simulink model "S_MTET_2RuleMa_MPPT_CONT_V1"  (R2017a)
settings: Solver=FixedStepDiscrete  StartTime=0.0  StopTime=10.0  RelTol=1e-3
values from neighbouring files (symbols this model uses):
  A = [0 (d-1)/L ... (first row only)    [M_MPPT_CONTROLLERS_SIM_V1.m]
undefined symbols (not defined in the file or in its folder): Down, GPTRIP1SEL, GPTRIP2SEL, TZ1, TZ2, Up
libraries: c2802xlib x3, c2806xlib x2, fuzblock x1
settings Model: ExtModeTrigDuration=8  Creator=dricl  LastModifiedBy=dricl
settings OptimizationCC: DefaultUnderspecifiedDataType=single  PassReuseOutputArgsAs=Individual arguments  MaxStackSize=512
settings DebuggingCC: ParameterTunabilityLossMsg=error
settings HardwareCC: ProdBitPerChar=16  ProdBitPerInt=16  ProdBitPerPointer=32  ProdBitPerSizeT=32  ProdBitPerPtrDiffT=32  ProdLargestAtomicInteger=Integer  ProdLargestAtomicFloat=None  ProdWordSize=16  ProdLongLongMode=on  ProdHWDeviceType=Texas Instruments->C2000
settings SFSimCC: MATLABDynamicMemAlloc=off
settings RTWCC: SystemTargetFile=ert.tlc  HardwareBoard=TI Piccolo F2806x  TLCOptions=-aInlineSetEventsForThisBaseRateFcn=TLC_FALSE -aSuppressMultiTaskScheduler=TLC_FALSE -aRateBasedStepFcn=1  TemplateMakefile=ert_default_tmf  Description=Embedded Coder  Toolchain=Texas Instruments Code Composer Studio v5 (C2000)  CodeExecutionProfiling=on  CodeProfilingSaveOptions=AllData  CodeProfilingInstrumentation=on
settings CodeAppCC: ForceParamTrailComments=on  IgnoreCustomStorageClasses=off  OperatorAnnotations=on  SimulinkDataObjDesc=on  SFDataObjDesc=on  MATLABFcnDesc=on  InsertBlockDesc=on  MATLABSourceComments=on
settings ERTTargetCC: CodeReplacementLibrary=TI C28x  MemSecPackage=tic2000demospkg  MemSecFuncExecute=code_ramfuncs

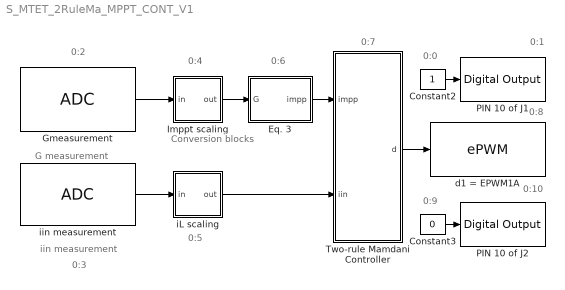
== system S_MTET_2RuleMa_MPPT_CONT_V1 ==
  note: iin measurement
  note: G measurement
  note: Conversion
      | blocks
  note: 0:2
  note: 0:3
  note: 0:4
  note: 0:6
  note: 0:5
  note: 0:7
  note: 0:10
  note: 0:9
  note: 0:0
  note: 0:1
  note: 0:8
  Constant2 : Constant  Priority=1  SampleTime=0.0002
  Constant3 : Constant  Priority=9  Value=0  SampleTime=0.0002
  Eq. 3 : Subsystem  Priority=5  TreatAsAtomicUnit=on
  Gmeasurement : c2802xlib/ADC  Priority=3  ADCModule=1  samplingMode=Single sample mode  ADCResolution=12-bit (Single-ended input)  useSOC1=SOC1  useSOC2=SOC0_SOC1  SOCAcquisitionWindow=7  SOCTriggerSource=ePWM1_ADCSOCA  SOCInterruptTrigger=No ADCINT  Ts=0.0002  dType=uint16  postInterrupt=off  interruptSel=ADCINT1  ADCINTContinuous=on  endma=off  chdma=1  blkParamProc=C2000  conv1=ADCINA1  conv2=ADCINA0 and ADCINB0  conv1_Type4=ADCIN0  conv2_Type4=ADCIN0 and ADCIN1
      settings: SourceProductName=Embedded Coder Support Package for Texas Instruments C2000 Processors
  Imppt scaling : Subsystem  Priority=5  TreatAsAtomicUnit=on
  PIN 10 of J1 : c2806xlib/Digital Output  Priority=2  GPIO_Number=GPIO32~GPIO39  GPIO_Bit0=on  GPIO_BIT0_Toggle=off  GPIO_Bit1=off  GPIO_BIT1_Toggle=off  GPIO_Bit2=off  GPIO_BIT2_Toggle=off  GPIO_Bit3=off  GPIO_BIT3_Toggle=off  GPIO_Bit4=off  GPIO_BIT4_Toggle=off  GPIO_Bit5=off  GPIO_BIT5_Toggle=off  GPIO_Bit6=off  GPIO_BIT6_Toggle=off  GPIO_Bit7=off  GPIO_BIT7_Toggle=off
      settings: SourceProductName=Embedded Coder Support Package for Texas Instruments C2000 Processors  SourceProductBaseCode=TIC2000
  PIN 10 of J2 : c2806xlib/Digital Output  Priority=10  GPIO_Number=GPIO32~GPIO39  GPIO_Bit0=on  GPIO_BIT0_Toggle=off  GPIO_Bit1=off  GPIO_BIT1_Toggle=off  GPIO_Bit2=off  GPIO_BIT2_Toggle=off  GPIO_Bit3=off  GPIO_BIT3_Toggle=off  GPIO_Bit4=off  GPIO_BIT4_Toggle=off  GPIO_Bit5=off  GPIO_BIT5_Toggle=off  GPIO_Bit6=off  GPIO_BIT6_Toggle=off  GPIO_Bit7=off  GPIO_BIT7_Toggle=off
      settings: SourceProductName=Embedded Coder Support Package for Texas Instruments C2000 Processors  SourceProductBaseCode=TIC2000
  Two-rule Mamdani Controller : Subsystem  Priority=7  TreatAsAtomicUnit=on
  d1 = EPWM1A : c2802xlib/ePWM  Priority=8  useModule=ePWM1  ePWMxLINKTBPRD=Not Linked  periodUnits=Clock cycles  timerSource=Specify via dialog  timerPeriod_clk=9000  timerPeriod_sec=0.0001  tbshadow=Counter equals to zero  countingMode=Up-Down  phaseActiveEnable=Disable  phaseDirection=Count down after sync  phaseActive=0  synchronizationEnable=off  dcaevt1Sync=off  dcbevt1Sync=off  synchronizationOption=Disable  clockPrescale=1  HSclockPrescale=1  enswap=off  ePWMxAStatus=on  ePWMxAactionLogic1=Do nothing  ePWMxAactionLogic2=Do nothing  ePWMxAactionLogic3=Clear  ePWMxAactionLogic4=Set  ePWMxAactionLogic5=Do nothing  ePWMxAactionLogic6=Do nothing  ePWMxALoadMode=Load on counter equals to zero (CTR=Zero)  ePWMxACSFenable=off  ePWMxACSFvalue=Forcing disable  ePWMxASFreload=Zero  ePWMxBStatus=off  ePWMxBactionLogic1=Set  ePWMxBactionLogic2=Clear  ePWMxBactionLogic3=Do nothing  ePWMxBactionLogic4=Do nothing  ePWMxBactionLogic5=Clear  ePWMxBactionLogic6=Set  ePWMxBLoadMode=Load on counter equals to zero (CTR=Zero)  ePWMxBCSFenable=off  ePWMxBCSFvalue=Forcing disable  ePWMxBSFreload=Zero  ePWNxBOutWay=off  ePWMxLINKCMPA=Not Linked  CMPAUnits=Clock cycles  CMPASource=Input port  CMPAValue_per=50  CMPAValue_clk=4500  enCMPAshadow=Counter equals to zero  ePWMxLINKCMPB=Not Linked  CMPBUnits=Clock cycles  CMPBSource=Specify via dialog  CMPBValue_per=50  CMPBValue_clk=4500  enCMPBshadow=Counter equals to zero  ePWMxLINKCMPC=Not Linked  CMPCUnits=Clock cycles  CMPCSource=Specify via dialog  CMPCValue_per=50  CMPCValue_clk=32000  enCMPCshadow=Counter equals to zero  ePWMxLINKCMPD=Not Linked  CMPDUnits=Clock cycles  CMPDSource=Specify via dialog  CMPDValue_per=50  CMPDValue_clk=32000  enCMPDshadow=Counter equals to zero  enableDBePWMxA=on  enableDBePWMxB=on  enhalfcycle=off  DBpolarity=Active high complementary (AHC)  DBedgeDelay=Positive  DBSource_ePWMxA=ePWMxA  DBSource_ePWMxB=ePWMxA  DBperiodSource=Specify via dialog  REDperiod=50  FEDperiod=50  adcstartModuleA=on  adcrequestEventA=First event  adcstartEventA=Counter equals to period (CTR=PRD)  adcstartEventA_type2=Digital Compare Module A Event 1 start of conversion (DCAEVT1.soc)  adcstartModuleB=off  adcrequestEventB=First event  adcstartEventB=Counter equals to zero (CTR=Zero)  adcstartEventB_type2=Counter equals to zero (CTR=Zero)  intEn=off  intPrd=First event  intSel=Counter equals to zero (CTR=Zero)  intSel_type2=Counter equals to zero (CTR=Zero)  hrpe=off  enHRPWM=off  HRPWM_LoadMode=Counter equals to period (CTR=PRD)  HRPWM_CTLMode=Duty or Period control mode  HRPWM_EDGMode=Both edge  hrpeb=off  enHRPWMB=off  HRPWM_LoadModeB=Counter equals to zero (CTR=ZERO)  HRPWM_CTLModeB=Duty or Period control mode  HRPWM_EDGModeB=Both edge  enSFO=on  enautoconv=on  chopperEnable=off  chopperFrequency=1  chopperFirstwidth=1  chopperDuty=12.5%  tripZonesource=Specify via dialog  tzselOSHT1=off  tzselOSHT2=off  tzselOSHT3=off  tzselOSHDCAEV1=off  tzselOSHDCBEV1=off  tzselCBC1=off  tzselCBC2=off  tzselCBC3=off  tzselCBCDCAEV2=off  tzselCBCDCBEV2=off  tzselOSHT4=off  tzselOSHT5=off  tzselOSHT6=off  tzselCBC4=off  tzselCBC5=off  tzselCBC6=off  enTzOstIntr=off  enTzCbcIntr=off  enTzDCAEVT1Intr=off  enTzDCAEVT2Intr=off  enTzDCBEVT1Intr=off  enTzDCBEVT2Intr=off  ePWMxAforced=No action  ePWMxBforced=No action  DCAEVT1forced=No action  DCBEVT1forced=No action  DCAEVT2forced=No action  DCBEVT2forced=No action  dcah=Trip Zone 1 input (TZ1)  dcal=Trip Zone 2 input (TZ2)  dcbh=Trip Zone 1 input (TZ1)  dcbl=Trip Zone 2 input (TZ2)  dcah_type2=GPTRIP1SEL/(TZ1)  dcal_type2=GPTRIP2SEL/(TZ2)  dcbh_type2=GPTRIP1SEL/(TZ1)  dcbl_type2=GPTRIP2SEL/(TZ2)  gendcaevt1=Event disabled  gendcaevt2=Event disabled  gendcbevt1=Event disabled  gendcbevt2=Event disabled  dcaevt1src=DCAEVT1 with sync  dcaevt2src=DCAEVT2 with sync  dcbevt1src=DCBEVT1 with sync  dcbevt2src=DCBEVT2 with sync  pulsesel=Counter equals to zero (CTR=Zero)  blankinv=off  blankoffset=0  blankwidth=0  evsrcsel=Filtered version of DCAEVT1 (DCAEVT1FILT)  encape=off  PwmType=C2000
      settings: SourceProductName=Embedded Coder Support Package for Texas Instruments C2000 Processors
  iL scaling : Subsystem  Priority=6  TreatAsAtomicUnit=on
  iin measurement : c2802xlib/ADC  Priority=4  ADCModule=1  samplingMode=Single sample mode  ADCResolution=12-bit (Single-ended input)  useSOC1=SOC2  useSOC2=SOC0_SOC1  SOCAcquisitionWindow=7  SOCTriggerSource=ePWM1_ADCSOCA  SOCInterruptTrigger=No ADCINT  Ts=0.0002  dType=uint16  postInterrupt=off  interruptSel=ADCINT1  ADCINTContinuous=on  endma=off  chdma=1  blkParamProc=C2000  conv1=ADCINA0  conv2=ADCINA0 and ADCINB0  conv1_Type4=ADCIN0  conv2_Type4=ADCIN0 and ADCIN1
      settings: SourceProductName=Embedded Coder Support Package for Texas Instruments C2000 Processors
  wires:
  iL scaling/1(out) -> Two-rule Mamdani Controller/2(iin)
  iin measurement/1 -> iL scaling/1(in)
  Constant2/1 -> PIN 10 of J1/1
  Constant3/1 -> PIN 10 of J2/1
  Two-rule Mamdani Controller/1(d) -> d1 = EPWM1A/1
  Imppt scaling/1(out) -> Eq. 3/1(G)
  Gmeasurement/1 -> Imppt scaling/1(in)
  Eq. 3/1(impp) -> Two-rule Mamdani Controller/1(impp)

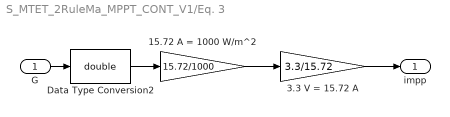
== system S_MTET_2RuleMa_MPPT_CONT_V1/Eq. 3 ==
  G : Inport
  " 15.72 A = 1000 W/m^2" : Gain  Gain=15.72/1000
  3.3 V = 15.72 A : Gain  Gain=3.3/15.72
  Data Type Conversion2 : DataTypeConversion  OutDataTypeStr=double
  impp : Outport
  wires:
  G/1 -> Data Type Conversion2/1
  " 15.72 A = 1000 W/m^2"/1 -> 3.3 V = 15.72 A/1
  3.3 V = 15.72 A/1 -> impp/1
  Data Type Conversion2/1 -> " 15.72 A = 1000 W/m^2"/1

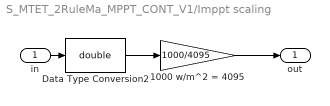
== system S_MTET_2RuleMa_MPPT_CONT_V1/Imppt scaling ==
  in : Inport
  1000 w/m^2 = 4095 : Gain  Gain=1000/4095
  Data Type Conversion2 : DataTypeConversion  OutDataTypeStr=double
  out : Outport
  wires:
  in/1 -> Data Type Conversion2/1
  Data Type Conversion2/1 -> 1000 w/m^2 = 4095/1
  1000 w/m^2 = 4095/1 -> out/1

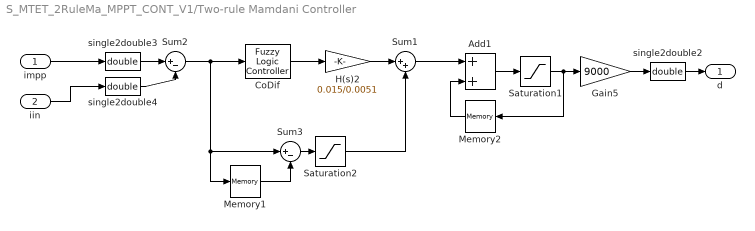
== system S_MTET_2RuleMa_MPPT_CONT_V1/Two-rule Mamdani Controller ==
  impp : Inport
  iin : Inport  Port=2
  Add1 : Sum
  CoDif : fuzblock/Fuzzy Logic  Controller  fis=['CoDif_Man_V2.fis']
  Gain5 : Gain  Gain=9000
  H(s)2 : Gain  Gain=0.015/0.0051
  Memory1 : Memory  InheritSampleTime=on
  Memory2 : Memory  InheritSampleTime=on
  Saturation1 : Saturate  UpperLimit=1  LowerLimit=0
  Saturation2 : Saturate  UpperLimit=0.03  LowerLimit=-0.03
  Sum1 : Sum  Inputs=|++
  Sum2 : Sum  Inputs=|+-
  Sum3 : Sum  Inputs=|+-
  single2double2 : DataTypeConversion  OutDataTypeStr=double
  single2double3 : DataTypeConversion  OutDataTypeStr=double
  single2double4 : DataTypeConversion  OutDataTypeStr=double
  d : Outport
  wires:
  impp/1 -> single2double3/1
  single2double2/1 -> d/1
  iin/1 -> single2double4/1
  Gain5/1 -> single2double2/1
  single2double3/1 -> Sum2/1
  single2double4/1 -> Sum2/2
  Sum2/1 -> CoDif/1, Sum3/1, Memory1/1
  Add1/1 -> Saturation1/1
  Saturation2/1 -> Sum1/2
  Memory1/1 -> Sum3/2
  Saturation1/1 -> Gain5/1, Memory2/1
  Memory2/1 -> Add1/2
  Sum1/1 -> Add1/1
  Sum3/1 -> Saturation2/1
  CoDif/1 -> H(s)2/1
  H(s)2/1 -> Sum1/1

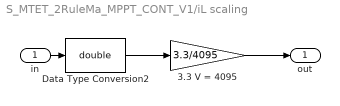
== system S_MTET_2RuleMa_MPPT_CONT_V1/iL scaling ==
  in : Inport
  3.3 V = 4095 : Gain  Gain=3.3/4095
  Data Type Conversion2 : DataTypeConversion  OutDataTypeStr=double
  out : Outport
  wires:
  in/1 -> Data Type Conversion2/1
  Data Type Conversion2/1 -> 3.3 V = 4095/1
  3.3 V = 4095/1 -> out/1
